simulink model "fft_dsp_lib"  (R2020a)
settings: Solver=VariableStepAuto  StartTime=0.0  StopTime=1  RelTol=1e-3
undefined symbols (not defined in the file): xc7vx485tffg1157
libraries: ModelComposer x3, simulink x2, dspxfrm3 x1, dspsrcs4 x1
settings Model: Creator=abehbood  LastModifiedBy=viswanad
settings HardwareCC: ProdBitPerPointer=32  ProdBitPerSizeT=32  ProdBitPerPtrDiffT=32  ProdLargestAtomicFloat=None  ProdIntDivRoundTo=Undefined  ProdEndianess=Unspecified  ProdWordSize=32  ProdHWDeviceType=ASIC/FPGA->ASIC/FPGA  TargetBitPerLong=64  TargetBitPerPointer=64  TargetBitPerSizeT=64  TargetBitPerPtrDiffT=64  TargetLongLongMode=on  TargetIntDivRoundTo=Zero  TargetEndianess=LittleEndian  TargetWordSize=64  TargetHWDeviceType=Custom Processor->MATLAB Host Computer  ProdEqTarget=off

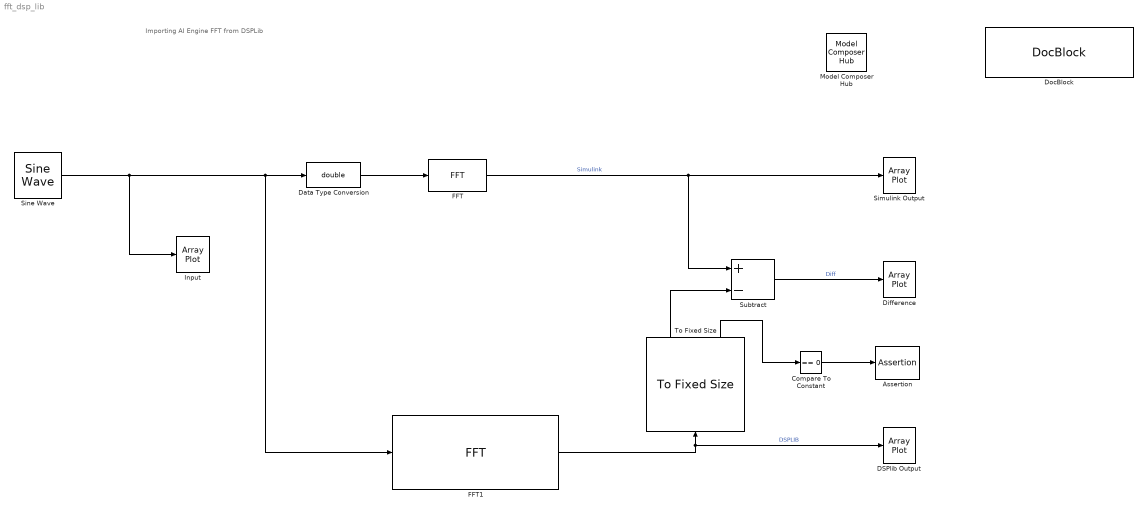
== system fft_dsp_lib ==
  note: Importing AI Engine FFT from DSPLib
  Assertion : Assertion
  Compare To Constant : simulink/Logic and Bit Operations/Compare To Constant  relop===  const=0  OutDataTypeStr=boolean
  DSPlib Output : ArrayPlot
  Data Type Conversion : DataTypeConversion  OutDataTypeStr=double
  Difference : ArrayPlot
  DocBlock : simulink/Model-Wide Utilities/DocBlock  DocumentType=Text  mask(DocBlock){}
      content=|
      | ///////////////////////////////////////////////////////////////////////////
      | // Copyright 2020 Xilinx
      | //
      | // Licensed under the Apache License, Version 2.0 (the "License");
      | // you may not use this file except in compliance with the License.
      | // You may obtain a copy of the License at
      | //
      | // http://www.apache.org/licenses/LICENSE-2.0
      | //
      | // Unless required by applicable law or agreed to in writing, software
      | // distributed under the License is distributed on an "AS IS" BASIS,
      | // WITHOUT WARRANTIES OR CONDITIONS OF ANY KIND, either express or implied.
      | // See the License for the specific language governing permissions and
      | // limitations under the License.
      | ///////////////////////////////////////////////////////////////////////////
      mask Display:
      | xmcDrawBlockIcon();
      | disp(['{\fontsize{10pt}(c) Copyright 2020' ' Xilinx, Inc.}\newline \newline '],'texmode','on');
      | disp('{\fontsize{10pt}Licensed under the Apache License 2.0}','texmode','on');
      | disp('\newline \newline \newline{\fontsize{10pt}Double Click for Copyright Notice}','texmode','on');
  FFT : dspxfrm3/FFT  FFTImplementation=Auto  CompMethod=Table lookup  TableOpt=NEW  TableOptActive=Speed  BitRevOrder=off  Normalize=off  InheritFFTLength=on  FFTLength=64  WrapInput=on  roundingMode=Floor  overflowMode=off  firstCoeffDataTypeStr=Inherit: Same word length as input  firstCoeffLastDataTypeStr=Inherit: Same word length as input  outputMin=[]  outputMax=[]
  FFT1 : ModelComposer/FFT  data_type=cint16  point_size=512  casc_length=1  shift_val=0  spec=meta_data_hl_fft.json
  Input : ArrayPlot
  Model Composer Hub : ModelComposer/Model Composer Hub  CodeGeneration=off  SubsystemName=dsplib_fft  TargetDirectory=./code  ExportType=AI Engines  IpVendor=xilinx.com  IpLibrary=hls  IpVersion=1.0  IpHWLanguage=Verilog  AieCompilerOptions={}  CreateTestbench=on  TestbenchStackSize=10  RunAieSim=on  AieSimTimeout=50000  RunAieSimProfiling=off  LaunchVitisAnalyzer=off  PlotOutput=off  RunX86Sim=off  X86SimTimeout=10  PlatformType=Not Specified  ProjDevice=xc7vx485tffg1157-1  ProjDevicePart=xc7vx485tffg1157-1  SamplePeriod=-1  ClockFrequency=200  DataPathParallelism=1
  Simulink Output : ArrayPlot
  Sine Wave : dspsrcs4/Sine Wave  Amplitude=64  Frequency=200  Phase=0  SampleMode=Discrete  OutComplex=Complex  CompMethod=Table lookup  TableSize=Speed  SampleTime=1/1000  SamplesPerFrame=512  ResetState=Restart at time zero  OutputFrames=off  dataType=Fixed-point  wordLen=16  udDataType=sfix(16)  fracBitsMode=User-defined  numFracBits=0  OutDataTypeStr=fixdt(1,16,0)  LastOutDataTypeStr=fixdt(1,16,0)
  Subtract : Sum  Inputs=+-
  To Fixed Size : ModelComposer/To Fixed Size  OutputSize=512  HasStatusOutput=on
  wires:
  FFT/1 -> Simulink Output/1, Subtract/1  "Simulink"
  FFT1/1 -> DSPlib Output/1, To Fixed Size/1  "DSPLIB"
  Subtract/1 -> Difference/1  "Diff"
  To Fixed Size/1 -> Subtract/2
  To Fixed Size/2 -> Compare To Constant/1
  Compare To Constant/1 -> Assertion/1
  Sine Wave/1 -> Input/1, Data Type Conversion/1, FFT1/1
  Data Type Conversion/1 -> FFT/1
